simulink model "single_cell_battery_phaseC_backup"  (R2025b)
settings: Solver=FixedStepDiscrete  StartTime=0.0  StopTime=1400  FixedStep=0.1  RelTol=1e-3
undefined symbols (not defined in the file): C2, Cc, Cs, DiscIntNeverNeededParam, I_test, inv_C1_2d_fixed, neg_inv_R1C1_2d_fixed, OCV_2d, Q_nom, R0_2d_fix, R1_2d, R2, Rcs, Rsa, soc_common, SoC_init, soc_ocv_common, T_amb, T_cell, T_init, temp_bp, temp_bp_ocv, Ts
settings Model: PacingRate=0.890000  Creator=mahad  LastModifiedBy=mahad
settings DataIOCC: SignalLogging=off  SaveTime=off
settings DebuggingCC: ReadBeforeWriteMsg=DisableAll  WriteAfterWriteMsg=DisableAll  WriteAfterReadMsg=DisableAll  MultiTaskDSMMsg=none
settings ModelReferenceCC: UpdateModelReferenceTargets=IfOutOfDate
settings SFSimCC: SFSimEcho=off

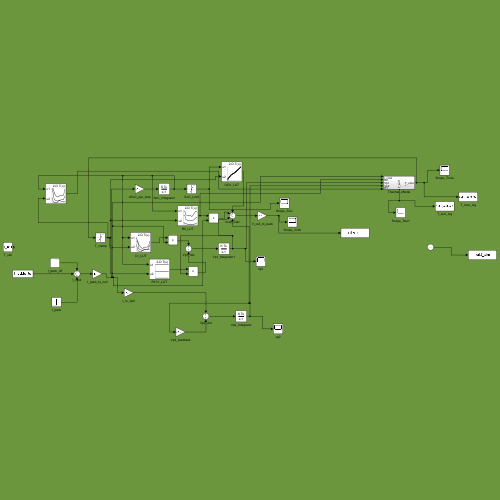
[thumbnail: Simulink's stored preview of the top-level diagram]
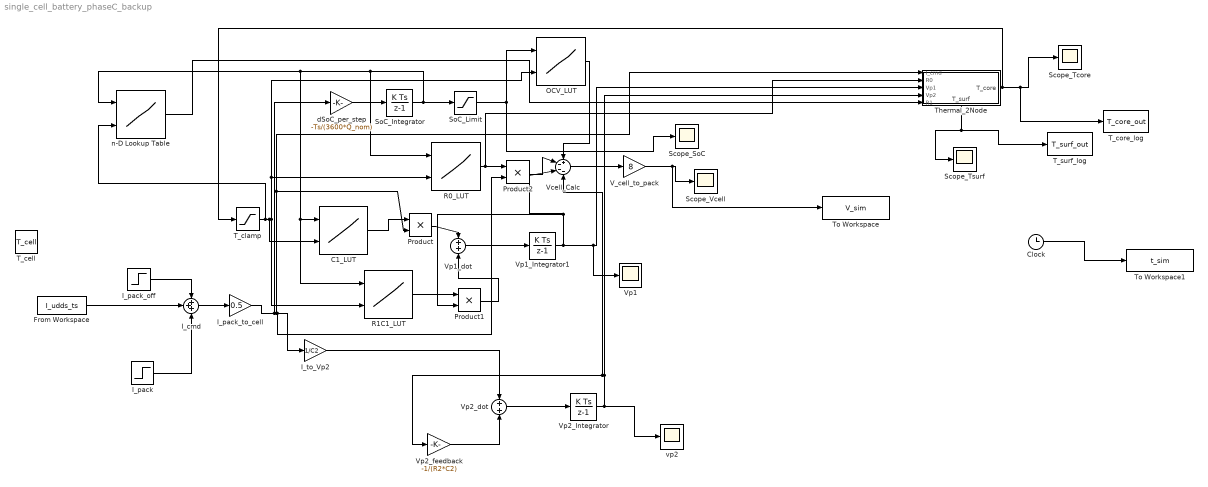
== system single_cell_battery_phaseC_backup ==
  " T_clamp" : Saturate  UpperLimit=25  LowerLimit=0
  C1_LUT : Lookup_n-D  BreakpointsForDimension1=soc_common  BreakpointsForDimension2=temp_bp  Table=inv_C1_2d_fixed  ExtrapMethod=Clip  InternalRulePriority=Speed  RndMeth=Simplest
      settings: InputPortMap=u0,u1
  Clock : Clock
  From Workspace : FromWorkspace  VariableName=I_udds_ts
  I_cmd : Sum  Inputs=+++
  I_pack : Step  Time=0  After=I_test  SampleTime=0.1
  I_pack_off : Step  Time=10  After=-I_test  SampleTime=0.1
  I_pack_to_cell : Gain  Gain=0.5
  I_to_Vp2 : Gain  Gain=1/C2
  OCV_LUT : Lookup_n-D  BreakpointsForDimension1=soc_ocv_common  BreakpointsForDimension2=temp_bp_ocv  BeginIndexSearchUsingPreviousIndexResult=on  Table=OCV_2d  ExtrapMethod=Clip  InternalRulePriority=Speed  RndMeth=Simplest
      settings: InputPortMap=u0,u1
  Product : Product
  Product1 : Product
  Product2 : Product
  R0_LUT : Lookup_n-D  BreakpointsForDimension1=soc_common  BreakpointsForDimension2=temp_bp  Table=R0_2d_fix  ExtrapMethod=Clip  InternalRulePriority=Speed  RndMeth=Simplest
      settings: InputPortMap=u0,u1
  R1C1_LUT : Lookup_n-D  BreakpointsForDimension1=soc_common  BreakpointsForDimension2=temp_bp  Table=neg_inv_R1C1_2d_fixed  ExtrapMethod=Clip  InternalRulePriority=Speed  RndMeth=Simplest
      settings: InputPortMap=u0,u1
  Scope_SoC : Scope
      settings: ActiveDisplayYMinimum=0.99939482470784613  ActiveDisplayYMaximum=1.0000672416991283  DataLoggingVariableName=SoC_log
  Scope_Tcore : Scope
      settings: ActiveDisplayYMinimum=24.999849468890503  ActiveDisplayYMaximum=25.001354779985498
  Scope_Tsurf : Scope
      settings: DataLoggingVariableName=ScopeData4
  Scope_Vcell : Scope
      settings: ActiveDisplayYMinimum=3.9024724539871976  ActiveDisplayYMaximum=4.18640131557632
  SoC_Integrator : DiscreteIntegrator  InitialCondition=SoC_init  SampleTime=0.1  ICPrevOutput=DiscIntNeverNeededParam  ICPrevScaledInput=DiscIntNeverNeededParam
  SoC_Limit : Saturate  UpperLimit=1  LowerLimit=0
  T_cell : Constant  Value=T_cell  SampleTime=-1
  T_core_log : ToWorkspace  VariableName=T_core_out  SaveFormat=Timeseries  SampleTime=-1
  T_surf_log : ToWorkspace  VariableName=T_surf_out  SaveFormat=Timeseries  SampleTime=-1
  Thermal_2Node : Subsystem
      settings: PortSchema="{\"entries\":[{\"content\":{\"sides\":[{\"content\":{\"connectorIds\":[\"In1\",\"In2\",\"In3\",\"In4\",\"In5\"]},\"type\":\"ConnectorPlacement.EquallySpacedRectSide\",\"uuid\":\"9beffa85-57a1-44dd-9942-a304dd24d92d\"},{\"content\":{\"connectorIds\":[\"Out1\"],\"side\":\"RIGHT\"},\"type\":\"ConnectorPlacement.EquallySpacedRectSide\",\"uuid\":\"e9ef47b7-1332-41b8-aa30-7951325d57fd\"},{\"content\":{\"side\":\"TOP\"},\"type\":\"ConnectorPlacement.EquallySpacedRectSide\",\"uuid\":\"60a3bd0d-bcfb-4657-8650-c1ed00b24a9b\"},{\"content\":{\"connectorIds\":[\"Out2\"],\"side\":\"BOTTOM\"},\"type\":\"ConnectorPlacement.EquallySpacedRectSide\",\"uuid\":\"dbfb8a93-4389-48f3-9eec-1566b5d198f7\"}]},\"type\":\"ConnectorPlacement.EquallySpacedConnector\",\"uuid\":\"32878aa3-c110-4f7b-a712-10cb32afef5e\"}],\"packageUris\":[\"http://schema.mathworks.com/mf0/Connector/R2020b\"],\"version\":\"1.0\"}"
  To Workspace : ToWorkspace  VariableName=V_sim  SampleTime=-1
  To Workspace1 : ToWorkspace  VariableName=t_sim  SampleTime=-1
  V_cell_to_pack : Gain  Gain=8
  Vcell_Calc : Sum  Inputs=+---
  Vp1 : Scope
      settings: ActiveDisplayYMinimum=-0.0028893234136200406  ActiveDisplayYMaximum=0.026003910722580369  DataLoggingVariableName=ScopeData2
  Vp1_Integrator1 : DiscreteIntegrator  SampleTime=0.1  ICPrevOutput=DiscIntNeverNeededParam  ICPrevScaledInput=DiscIntNeverNeededParam
  Vp1_dot : Sum
  Vp2_Integrator : DiscreteIntegrator  SampleTime=0.1  ICPrevOutput=DiscIntNeverNeededParam  ICPrevScaledInput=DiscIntNeverNeededParam
  Vp2_dot : Sum
  Vp2_feedback : Gain  Gain=-1/(R2*C2)
  dSoC_per_step : Gain  Gain=-Ts/(3600*Q_nom)
  n-D Lookup Table : Lookup_n-D  BreakpointsForDimension1=soc_common  BreakpointsForDimension2=temp_bp  BreakpointsForDimension3=[5, 7]  Table=R1_2d  ExtrapMethod=Clip  InternalRulePriority=Speed  RndMeth=Simplest
      settings: InputPortMap=u0,u1
  vp2 : Scope
      settings: ActiveDisplayYMinimum=-0.00021306760205067724  ActiveDisplayYMaximum=0.0019176084184560956  DataLoggingVariableName=ScopeData3
  wires:
  dSoC_per_step/1 -> SoC_Integrator/1
  SoC_Integrator/1 -> n-D Lookup Table/1, R1C1_LUT/1, C1_LUT/1, R0_LUT/1, SoC_Limit/1
  SoC_Limit/1 -> OCV_LUT/1, Scope_SoC/1
  OCV_LUT/1 -> Vcell_Calc/1
  Vp1_Integrator1/1 -> Thermal_2Node/3(Vp1), Vp1/1, Product1/2, Vcell_Calc/3
  Vp1_dot/1 -> Vp1_Integrator1/1
  Vp2_dot/1 -> Vp2_Integrator/1
  Vp2_Integrator/1 -> Thermal_2Node/4(Vp2), Vcell_Calc/4, Vp2_feedback/1, vp2/1
  I_to_Vp2/1 -> Vp2_dot/1
  Vp2_feedback/1 -> Vp2_dot/2
  Clock/1 -> To Workspace1/1
  C1_LUT/1 -> Product/1
  Product/1 -> Vp1_dot/1
  R1C1_LUT/1 -> Product1/1
  Product1/1 -> Vp1_dot/2
  R0_LUT/1 -> Thermal_2Node/2(R0), Product2/1
  Product2/1 -> Vcell_Calc/2
  I_pack_off/1 -> I_cmd/1
  Thermal_2Node/1(T_core) -> " T_clamp"/1, T_core_log/1, Scope_Tcore/1
  Thermal_2Node/2(T_surf) -> T_surf_log/1, Scope_Tsurf/1
  " T_clamp"/1 -> n-D Lookup Table/2, C1_LUT/2, R0_LUT/2, OCV_LUT/2, R1C1_LUT/2
  n-D Lookup Table/1 -> Thermal_2Node/5(R1)
  From Workspace/1 -> I_cmd/2
  I_pack/1 -> I_cmd/3
  I_cmd/1 -> I_pack_to_cell/1
  I_pack_to_cell/1 -> dSoC_per_step/1, Thermal_2Node/1(I_cmd), Product/2, Product2/2, I_to_Vp2/1
  Vcell_Calc/1 -> V_cell_to_pack/1
  V_cell_to_pack/1 -> To Workspace/1, Scope_Vcell/1

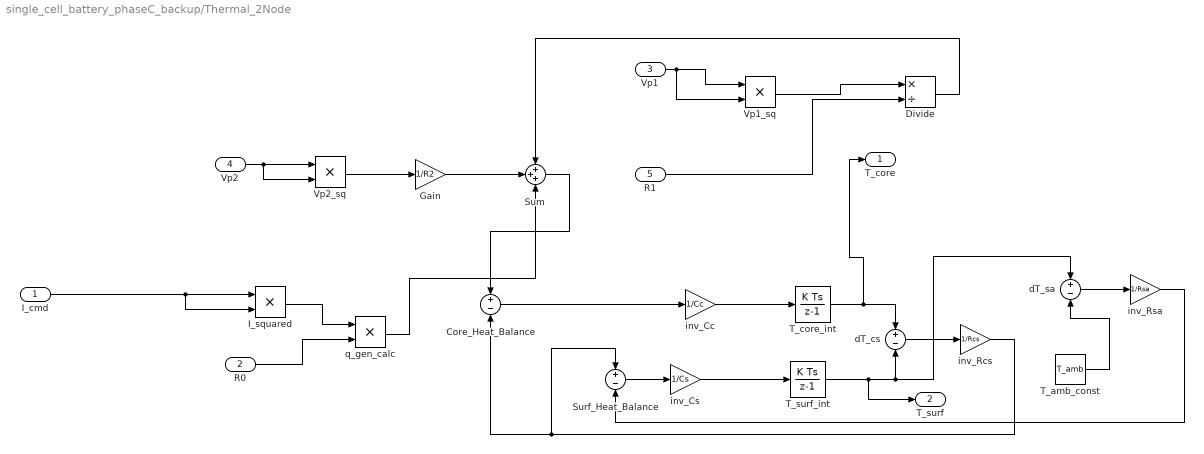
== system single_cell_battery_phaseC_backup/Thermal_2Node ==
  I_cmd : Inport
  R0 : Inport  Port=2
  Vp1 : Inport  Port=3
  Vp2 : Inport  Port=4
  R1 : Inport  Port=5
  Core_Heat_Balance : Sum  Inputs=+-
  Divide : Product  Inputs=*/
  Gain : Gain  Gain=1/R2
  I_squared : Product  Inputs=**
  Sum : Sum  Inputs=+++
  Surf_Heat_Balance : Sum  Inputs=+-
  T_amb_const : Constant  Value=T_amb
  T_core_int : DiscreteIntegrator  InitialCondition=T_init  SampleTime=0.1  ICPrevOutput=DiscIntNeverNeededParam  ICPrevScaledInput=DiscIntNeverNeededParam
  T_surf_int : DiscreteIntegrator  InitialCondition=T_init  SampleTime=0.1  ICPrevOutput=DiscIntNeverNeededParam  ICPrevScaledInput=DiscIntNeverNeededParam
  Vp1_sq : Product
  Vp2_sq : Product
  dT_cs : Sum  Inputs=+-
  dT_sa : Sum  Inputs=+-
  inv_Cc : Gain  Gain=1/Cc
  inv_Cs : Gain  Gain=1/Cs
  inv_Rcs : Gain  Gain=1/Rcs
  inv_Rsa : Gain  Gain=1/Rsa
  q_gen_calc : Product  Inputs=**
  T_core : Outport
  T_surf : Outport  Port=2
  wires:
  I_cmd/1 -> I_squared/2, I_squared/1
  I_squared/1 -> q_gen_calc/1
  R0/1 -> q_gen_calc/2
  Core_Heat_Balance/1 -> inv_Cc/1
  inv_Cc/1 -> T_core_int/1
  Surf_Heat_Balance/1 -> inv_Cs/1
  inv_Cs/1 -> T_surf_int/1
  T_surf_int/1 -> T_surf/1, dT_sa/1, dT_cs/2
  T_core_int/1 -> T_core/1, dT_cs/1
  dT_cs/1 -> inv_Rcs/1
  inv_Rcs/1 -> Core_Heat_Balance/2, Surf_Heat_Balance/1
  T_amb_const/1 -> dT_sa/2
  dT_sa/1 -> inv_Rsa/1
  inv_Rsa/1 -> Surf_Heat_Balance/2
  Vp1/1 -> Vp1_sq/2, Vp1_sq/1
  Vp1_sq/1 -> Divide/1
  R1/1 -> Divide/2
  Vp2/1 -> Vp2_sq/2, Vp2_sq/1
  Vp2_sq/1 -> Gain/1
  q_gen_calc/1 -> Sum/3
  Divide/1 -> Sum/1
  Gain/1 -> Sum/2
  Sum/1 -> Core_Heat_Balance/1
